simulink model "IP_LQG_PCI6221_2015a"  (R2015b)
settings: Solver=ode5  StartTime=0.0  StopTime=30  RelTol=1e-3
values from neighbouring files (symbols this model uses):
  A_aug = [0 0 0 0 0 1 1 -0.0174048595758 0 -0.0173759205618 -232.025201375 0 ... (36 elements, 6x6)]    [lqg-integrador-standard-no-perturb.mat]    (also in lqg-integrador-standard-perturb-2.mat; lqg-integrador-standard-perturb.mat; lqg-integrator-pertu.mat; lqg-integrator.mat)
  ALPHA_MAX = 1.57079632679    [lqg-integrador-standard-no-perturb.mat]    (also in lqg-integrador-standard-perturb-2.mat; lqg-integrador-standard-perturb.mat; lqg-integrator-pertu.mat; lqg-integrator.mat)
  B_aug = [0 0 0 0 333.33674813 0]    [lqg-integrador-standard-no-perturb.mat]    (also in lqg-integrador-standard-perturb-2.mat; lqg-integrador-standard-perturb.mat; lqg-integrator-pertu.mat; lqg-integrator.mat)
  BETA_MAX = 0.261799387799    [lqg-integrador-standard-no-perturb.mat]    (also in lqg-integrador-standard-perturb-2.mat; lqg-integrador-standard-perturb.mat; lqg-integrator-pertu.mat; lqg-integrator.mat)
  C_aug = [1  0  0  0  0  0; 0  0  1  0  0  0]    [lqg-integrador-standard-no-perturb.mat]    (also in lqg-integrador-standard-perturb-2.mat; lqg-integrador-standard-perturb.mat; lqg-integrator-pertu.mat; lqg-integrator.mat)
  K = [-35.2521787893 -12.8325964614 96.6145862802 14.5036883731 0.122144859777 -10]    [lqg-integrador-standard-no-perturb.mat]    (also in lqg-integrador-standard-perturb-2.mat; lqg-integrador-standard-perturb.mat; lqg-integrator-pertu.mat = [-112.979481029 -36.3845922499 259.380209538 39.3388003244 0; lqg-integrator.mat = [-112.979481029 -36.3845922499 259.380209538 39.3388003244 0)
  L_aug = [1811.88041562  -0.0198011616491; 52.1454441199  -25.0448593517; -0.0198011616491  1813.26844834; -46.7372993057  2568.05805966; -15.8003227076  12.5918014891; 1  0]    [lqg-integrador-standard-no-perturb.mat]    (also in lqg-integrador-standard-perturb-2.mat; lqg-integrador-standard-perturb.mat; lqg-integrator-pertu.mat; lqg-integrator.mat)
  TIME_DELAY = 6    [lqg-integrador-standard-no-perturb.mat]    (also in lqg-integrador-standard-perturb-2.mat; lqg-integrador-standard-perturb.mat; lqg-integrator-pertu.mat; lqg-integrator.mat)
  Ts = 0.001    [lqg-integrador-standard-no-perturb.mat]    (also in lqg-integrador-standard-perturb-2.mat; lqg-integrador-standard-perturb.mat; lqg-integrator-pertu.mat; lqg-integrator.mat)
  V_MAX = 5    [lqg-integrador-standard-no-perturb.mat]    (also in lqg-integrador-standard-perturb-2.mat; lqg-integrador-standard-perturb.mat; lqg-integrator-pertu.mat; lqg-integrator.mat)
  V_MIN = -5    [lqg-integrador-standard-no-perturb.mat]    (also in lqg-integrador-standard-perturb-2.mat; lqg-integrador-standard-perturb.mat; lqg-integrator-pertu.mat; lqg-integrator.mat)
undefined symbols (not defined in the file or in its folder): National_Instruments, PCI
libraries: sldrtlib x3, simulink x2
settings Model: SimulationMode=external  ExtModeTrigDuration=100000  Creator=Alunos  LastModifiedBy=CMNO
settings DataIOCC: SaveFormat=Array
settings HardwareCC: ProdBitPerPointer=32  ProdLargestAtomicFloat=None  ProdWordSize=32  ProdHWDeviceType=Intel->x86/Pentium  TargetIntDivRoundTo=Zero  TargetEndianess=LittleEndian  TargetHWDeviceType=Intel->x86/Pentium
settings RTWCC: SystemTargetFile=sldrt.tlc  TemplateMakefile=sldrt.tmf  Description=Simulink Desktop Real-Time  RTWCompilerOptimization=on
settings CodeAppCC: MaxIdLength=95
settings SimulinkDesktopRealTimeCC: TargetPreCompLibLocation=C:\Program Files\MATLAB\R2015b\toolbox\sldrt\lib\win32  TargetLangStandard=C89/C90 (ANSI)  SupportVariableSizeSignals=off
settings ConfigComp: CovHtmlReporting=off  CovModelRefEnable=Off

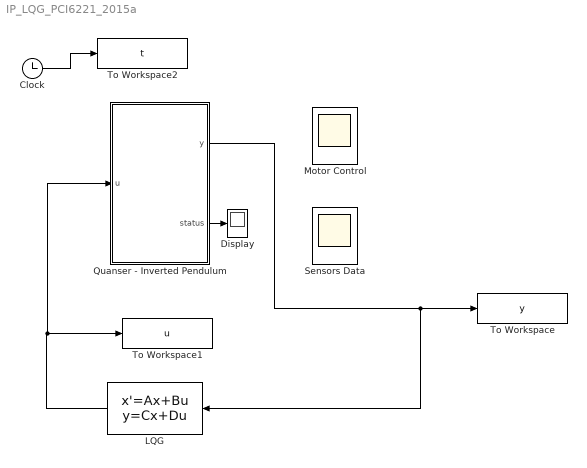
== system IP_LQG_PCI6221_2015a ==
  Clock : Clock
  Display : Display
  LQG : StateSpace  A=A_aug - B_aug * K - L_aug * C_aug  B=L_aug  C=-K  D=zeros(1,2)  X0=zeros(6,1)
  Motor Control : Scope
      settings: Floating=on
  Quanser - Inverted Pendulum : Subsystem
      mask Display: image('IP_QUANSER.jpg');
  Sensors Data : Scope
      settings: Floating=on
  To Workspace : ToWorkspace  VariableName=y  SaveFormat=Structure With Time  SampleTime=-1
  To Workspace1 : ToWorkspace  VariableName=u  SaveFormat=Structure With Time  SampleTime=-1
  To Workspace2 : ToWorkspace  VariableName=t  SaveFormat=Structure With Time  SampleTime=-1
  wires:
  Quanser - Inverted Pendulum/1(y) -> LQG/1, To Workspace/1
  Quanser - Inverted Pendulum/2(status) -> Display/1
  LQG/1 -> Quanser - Inverted Pendulum/1(u), To Workspace1/1
  Clock/1 -> To Workspace2/1

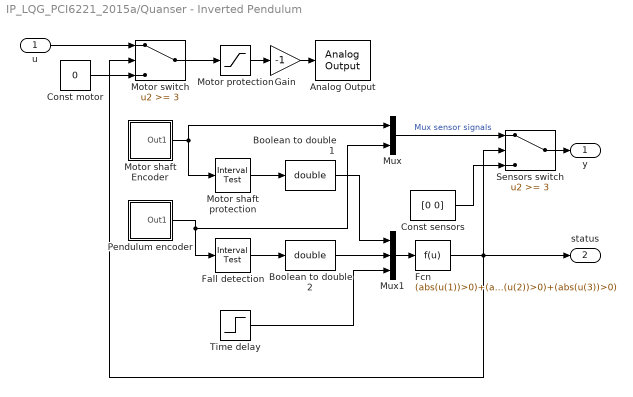
== system IP_LQG_PCI6221_2015a/Quanser - Inverted Pendulum ==
  u : Inport
  Analog Output : sldrtlib/Analog Output  SampleTime=Ts  MaxMissedTicks=10  ShowMissedTicks=off  YieldWhenWaiting=off  DrvName=National_Instruments/PCI-6221  DrvAddress=4294967295  DrvOptions=[0 0 0 2 2]  Channels=1  RangeMode=1  VoltRange=1  InitialValue=0  FinalValue=0
      settings: AttributesFormatString=National Instruments\nPCI-6221 [auto]
  Boolean to double 1 : DataTypeConversion  OutDataTypeStr=double
  Boolean to double 2 : DataTypeConversion  OutDataTypeStr=double
  Const motor : Constant  Value=0
  Const sensors : Constant  Value=[0 0]
  Fall detection : simulink/Logic and Bit Operations/Interval Test  IntervalClosedRight=on  uplimit=BETA_MAX  IntervalClosedLeft=on  lowlimit=-BETA_MAX  OutDataTypeStr=uint8
  Fcn : Fcn  Expr=(abs(u(1))>0)+(abs(u(2))>0)+(abs(u(3))>0)
  Gain : Gain  Gain=-1
  Motor protection : Saturate  UpperLimit=V_MAX  LowerLimit=V_MIN
  Motor shaft Encoder : Subsystem
  Motor shaft protection : simulink/Logic and Bit Operations/Interval Test  IntervalClosedRight=on  uplimit=ALPHA_MAX  IntervalClosedLeft=on  lowlimit=-ALPHA_MAX  OutDataTypeStr=uint8
  Motor switch : Switch  Threshold=3
  Mux : Mux  Inputs=2
  Mux1 : Mux  Inputs=3
  Pendulum encoder : Subsystem
  Sensors switch : Switch  Threshold=3
  Time delay : Step  Time=TIME_DELAY  SampleTime=0
  y : Outport
  status : Outport  Port=2
  wires:
  u/1 -> Motor switch/1
  Motor switch/1 -> Motor protection/1
  Const motor/1 -> Motor switch/3
  Motor shaft Encoder/1(Out1) -> Mux/1, Motor shaft protection/1
  Pendulum encoder/1(Out1) -> Fall detection/1, Mux/2
  Mux1/1 -> Fcn/1
  Fcn/1 -> Sensors switch/2, status/1, Motor switch/2
  Time delay/1 -> Mux1/3
  Fall detection/1 -> Boolean to double 2/1
  Boolean to double 2/1 -> Mux1/2
  Motor shaft protection/1 -> Boolean to double 1/1
  Boolean to double 1/1 -> Mux1/1
  Const sensors/1 -> Sensors switch/3
  Mux/1 -> Sensors switch/1  "Mux sensor signals"
  Sensors switch/1 -> y/1
  Gain/1 -> Analog Output/1
  Motor protection/1 -> Gain/1

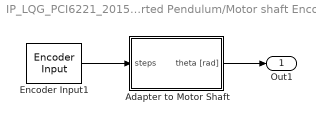
== system IP_LQG_PCI6221_2015a/Quanser - Inverted Pendulum/Motor shaft Encoder ==
  Adapter to Motor Shaft : Subsystem
  Encoder Input1 : sldrtlib/Encoder Input  SampleTime=Ts  MaxMissedTicks=inf  ShowMissedTicks=off  YieldWhenWaiting=off  DrvName=National_Instruments/PCI-6221  DrvAddress=4294967295  DrvOptions=[0 0 0 2 2]  Channels=1  QuadMode=3  IndexPulse=2  InputFilter=Inf  DataType=1
      settings: AttributesFormatString=National Instruments\nPCI-6221 [auto]
  Out1 : Outport
  wires:
  Encoder Input1/1 -> Adapter to Motor Shaft/1(steps)
  Adapter to Motor Shaft/1(theta [rad]) -> Out1/1

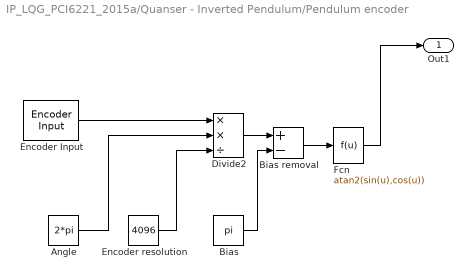
== system IP_LQG_PCI6221_2015a/Quanser - Inverted Pendulum/Pendulum encoder ==
  Angle : Constant  Value=2*pi
  Bias : Constant  Value=pi
  Bias removal : Sum  Inputs=+-
  Divide2 : Product  Inputs=**/
  Encoder resolution : Constant  Value=4096
  Encoder Input : sldrtlib/Encoder Input  SampleTime=Ts  MaxMissedTicks=inf  ShowMissedTicks=off  YieldWhenWaiting=off  DrvName=National_Instruments/PCI-6221  DrvAddress=4294967295  DrvOptions=[0 0 0 2 2]  Channels=2  QuadMode=3  IndexPulse=2  InputFilter=Inf  DataType=1
      settings: AttributesFormatString=National Instruments\nPCI-6221 [auto]
  Fcn : Fcn  Expr=atan2(sin(u),cos(u))
  Out1 : Outport
  wires:
  Bias/1 -> Bias removal/2
  Encoder resolution/1 -> Divide2/3
  Divide2/1 -> Bias removal/1
  Fcn/1 -> Out1/1
  Encoder Input/1 -> Divide2/1
  Bias removal/1 -> Fcn/1
  Angle/1 -> Divide2/2

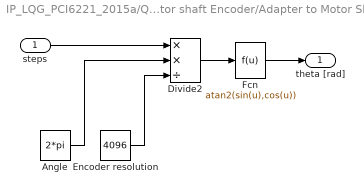
== system IP_LQG_PCI6221_2015a/Quanser - Inverted Pendulum/Motor shaft Encoder/Adapter to Motor Shaft ==
  steps : Inport
  Angle : Constant  Value=2*pi
  Divide2 : Product  Inputs=**/
  Encoder resolution : Constant  Value=4096
  Fcn : Fcn  Expr=atan2(sin(u),cos(u))
  theta [rad] : Outport
  wires:
  Angle/1 -> Divide2/2
  Encoder resolution/1 -> Divide2/3
  steps/1 -> Divide2/1
  Divide2/1 -> Fcn/1
  Fcn/1 -> theta [rad]/1
